simulink model "grading"  (R2016b)
settings: Solver=ode8  StartTime=0.0  StopTime=10.0  RelTol=1e-3
settings Model: Creator=Radwa  LastModifiedBy=Radwa

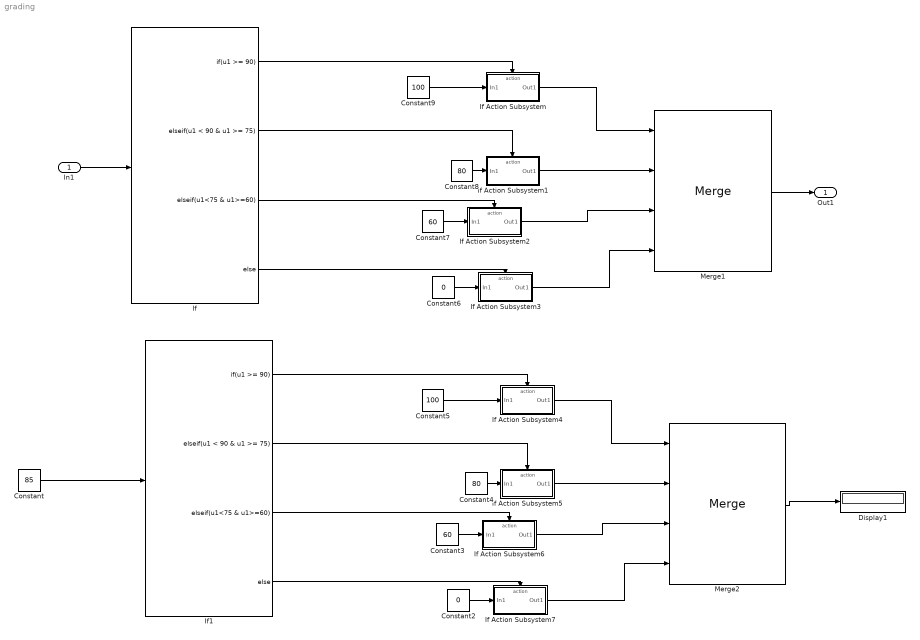
== system grading ==
  In1 : Inport
  Constant : Constant  Value=85
  Constant2 : Constant  Value=0
  Constant3 : Constant  Value=60
  Constant4 : Constant  Value=80
  Constant5 : Constant  Value=100
  Constant6 : Constant  Value=0
  Constant7 : Constant  Value=60
  Constant8 : Constant  Value=80
  Constant9 : Constant  Value=100
  Display1 : Display
  If : If  IfExpression=u1 >= 90  ElseIfExpressions=u1 < 90 & u1 >= 75, u1<75 & u1>=60
  If Action Subsystem : Subsystem  TreatAsAtomicUnit=on
  If Action Subsystem1 : Subsystem  TreatAsAtomicUnit=on
  If Action Subsystem2 : Subsystem  TreatAsAtomicUnit=on
  If Action Subsystem3 : Subsystem  TreatAsAtomicUnit=on
  If Action Subsystem4 : Subsystem  TreatAsAtomicUnit=on
  If Action Subsystem5 : Subsystem  TreatAsAtomicUnit=on
  If Action Subsystem6 : Subsystem  TreatAsAtomicUnit=on
  If Action Subsystem7 : Subsystem  TreatAsAtomicUnit=on
  If1 : If  IfExpression=u1 >= 90  ElseIfExpressions=u1 < 90 & u1 >= 75, u1<75 & u1>=60
  Merge1 : Merge  Inputs=4
  Merge2 : Merge  Inputs=4
  Out1 : Outport
  wires:
  Merge1/1 -> Out1/1
  If/1 -> If Action Subsystem/Action
  If Action Subsystem/1(Out1) -> Merge1/1
  Constant9/1 -> If Action Subsystem/1(In1)
  If Action Subsystem3/1(Out1) -> Merge1/4
  If Action Subsystem2/1(Out1) -> Merge1/3
  If Action Subsystem1/1(Out1) -> Merge1/2
  Constant8/1 -> If Action Subsystem1/1(In1)
  Constant7/1 -> If Action Subsystem2/1(In1)
  Constant6/1 -> If Action Subsystem3/1(In1)
  If/4 -> If Action Subsystem3/Action
  If/2 -> If Action Subsystem1/Action
  If/3 -> If Action Subsystem2/Action
  In1/1 -> If/1
  Merge2/1 -> Display1/1
  If1/1 -> If Action Subsystem4/Action
  If Action Subsystem4/1(Out1) -> Merge2/1
  Constant5/1 -> If Action Subsystem4/1(In1)
  If Action Subsystem7/1(Out1) -> Merge2/4
  If Action Subsystem6/1(Out1) -> Merge2/3
  If Action Subsystem5/1(Out1) -> Merge2/2
  Constant4/1 -> If Action Subsystem5/1(In1)
  Constant3/1 -> If Action Subsystem6/1(In1)
  Constant2/1 -> If Action Subsystem7/1(In1)
  If1/4 -> If Action Subsystem7/Action
  If1/2 -> If Action Subsystem5/Action
  If1/3 -> If Action Subsystem6/Action
  Constant/1 -> If1/1

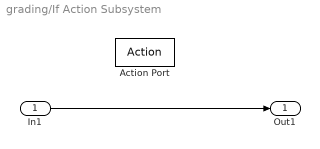
== system grading/If Action Subsystem ==
  In1 : Inport
  Action Port : ActionPort  ActionType=then
  Out1 : Outport
  wires:
  In1/1 -> Out1/1

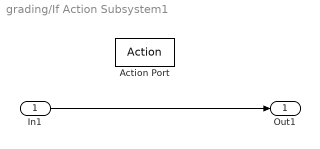
== system grading/If Action Subsystem1 ==
  In1 : Inport
  Action Port : ActionPort  ActionType=elseif
  Out1 : Outport
  wires:
  In1/1 -> Out1/1

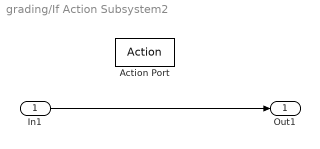
== system grading/If Action Subsystem2 ==
  In1 : Inport
  Action Port : ActionPort  ActionType=elseif
  Out1 : Outport
  wires:
  In1/1 -> Out1/1

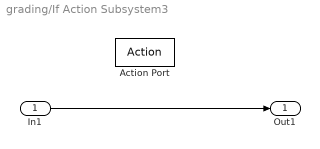
== system grading/If Action Subsystem3 ==
  In1 : Inport
  Action Port : ActionPort  ActionType=else
  Out1 : Outport
  wires:
  In1/1 -> Out1/1

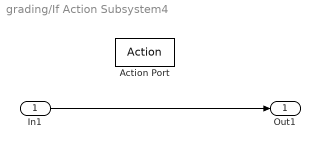
== system grading/If Action Subsystem4 ==
  In1 : Inport
  Action Port : ActionPort  ActionType=then
  Out1 : Outport
  wires:
  In1/1 -> Out1/1

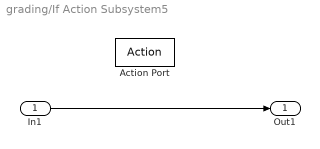
== system grading/If Action Subsystem5 ==
  In1 : Inport
  Action Port : ActionPort  ActionType=elseif
  Out1 : Outport
  wires:
  In1/1 -> Out1/1

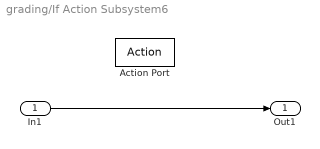
== system grading/If Action Subsystem6 ==
  In1 : Inport
  Action Port : ActionPort  ActionType=elseif
  Out1 : Outport
  wires:
  In1/1 -> Out1/1

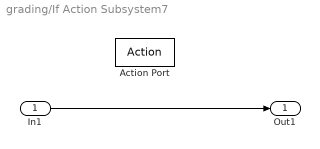
== system grading/If Action Subsystem7 ==
  In1 : Inport
  Action Port : ActionPort  ActionType=else
  Out1 : Outport
  wires:
  In1/1 -> Out1/1
